simulink model "untitled"  (R2014a)
settings: Solver=ode45  StartTime=0.0  StopTime=100  RelTol=1e-3
settings Model: Creator=York  LastModifiedBy=York

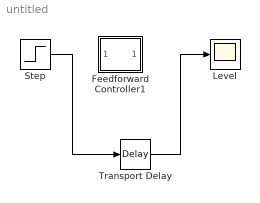
== system untitled ==
  Feedforward Controller1 : Subsystem  mask(feedforward Controller){K=1, T1=10, T2=5, t=5}
      mask prompts: K "Kffl:"; T1 "Tlead:"; T2 "Tlag:"; t "tff:"
      mask Display: disp('Gff(s)')
  Level : Scope
      settings: TickLabels=on  TimeRange=200  YMin=-2.000000  YMax=2.000000  SaveName=ScopeData3
  Step : Step  Time=0  SampleTime=0
  Transport Delay : TransportDelay  DelayTime=4
  wires:
  Step/1 -> Transport Delay/1
  Transport Delay/1 -> Level/1

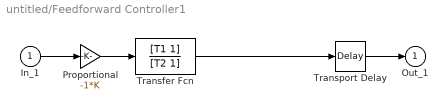
== system untitled/Feedforward Controller1 ==
  In_1 : Inport
  Proportional : Gain  Gain=-1*K  SaturateOnIntegerOverflow=on  OutDataTypeStr=Inherit: Same as input  ParamDataTypeStr=Inherit: Same as input
  Transfer Fcn : TransferFcn  Numerator=[T1 1]  Denominator=[T2 1]
  Transport Delay : TransportDelay  DelayTime=t
  Out_1 : Outport  InitialOutput=0
  wires:
  In_1/1 -> Proportional/1
  Proportional/1 -> Transfer Fcn/1
  Transfer Fcn/1 -> Transport Delay/1
  Transport Delay/1 -> Out_1/1
